simulink model "commrfsatlink"  (R2025a)
settings: Solver=VariableStepDiscrete  StartTime=0.0  StopTime=1  RelTol=1e-3  EnableMultiTasking=on
PreLoadFcn:
  | commrfsatlink_mask(1, 2, 1, 1, 1, ...
  |     0, 0, 0, 35600, 4000,[.4 .4],4,6,0,'No ADC');
values from neighbouring files (symbols this model uses):
  rfSatSourceSamplesPerSymbol = 400    [commrfsatlink_mask.m]
  rfSatSourceSampleTime = 1e-5    (= 1e-05)    [commrfsatlink_mask.m]
undefined symbols (not defined in the file or in its folder): paramRFSatLink, QAM
libraries: commrflib2 x6, dspsigops x3, commrfcorlib x2, dspsolvers x2, simulink x2, commfilt2 x2, commdigbbndam3 x2, commdemoslib x1, impairlib x1, commsink2 x1, commrandsrc3 x1, commsync2 x1
Description:
  | RF Satellite Link
settings Model: FPTRunName=Active  ExtModeAutoUpdateStatusClock=off  Creator=The MathWorks, Inc.  LastModifiedBy=daniel
settings SolverCC: AlgebraicLoopSolver=TrustRegion
settings DataIOCC: LimitDataPoints=on  SaveFormat=Array  SaveOutput=off  SaveTime=off  ReturnWorkspaceOutputs=off  SignalLoggingName=satlinkSigsOut
settings OptimizationCC: OptimizeBlockIOStorage=off  BufferReuse=off  GlobalBufferReuse=off  ExpressionFolding=off  ExpressionDepthLimit=2147483647.0  LocalBlockOutputs=off  InitFltsAndDblsToZero=on  EfficientMapNaN2IntZero=off  LifeSpan=inf  BufferReusableBoundary=off  OptimizeDataStoreBuffers=off  BusAssignmentInplaceUpdate=off
settings DebuggingCC: SaveWithParameterizedLinksMsg=none  UnderspecifiedInitializationDetection=Classic  MergeDetectMultiDrivingBlocksExec=none  CheckExecutionContextPreStartOutputMsg=on  SignalResolutionControl=TryResolveAllWithWarning  InheritedTsInSrcMsg=none  MultiTaskDSMMsg=warning  MultiTaskCondExecSysMsg=none  SigSpecEnsureSampleTimeMsg=none  FcnCallInpInsideContextMsg=warning  UnconnectedInputMsg=warning  UnconnectedOutputMsg=warning  UnconnectedLineMsg=warning  BusObjectLabelMismatch=none  AllowSymbolicDim=off  StateNameClashWarn=warning  PregeneratedLibrarySubsystemCodeDiagnostic=none  SFUnexpectedBacktrackingDiag=warning  SFNoUnconditionalDefaultTransitionDiag=warning  SFExecutionAtInitializationDiag=none  ArithmeticOperatorsInVariantConditions=warning
settings HardwareCC: ProdBitPerPointer=32.0  ProdLargestAtomicFloat=None  ProdIntDivRoundTo=Undefined  ProdEndianess=Unspecified  ProdWordSize=32.0  ProdHWDeviceType=32-bit Generic  TargetUnknown=on
settings ModelReferenceCC: UpdateModelReferenceTargets=IfOutOfDate  EnableRefExpFcnMdlSchedulingChecks=on  PropagateSignalLabelsOutOfModel=off
settings SFSimCC: SimUseLocalCustomCode=off  CustomCodeUndefinedFunction=UseInterfaceOnly
settings RTWCC: RTWUseLocalCustomCode=off  GPUComputeCapability=3.5
settings CodeAppCC: StateflowObjectComments=on
settings GRTTargetCC: TargetFcnLib=ansi_tfl_tmw.mat  TargetLangStandard=C89/C90 (ANSI)  CombineOutputUpdateFcns=off  GRTInterface=on
settings ConfigComp: CovMetricSettings=dw  CovSaveCumulativeToWorkspaceVar=on  CovSaveSingleToWorkspaceVar=on  CovExternalEMLEnable=off  CovSFcnEnable=off

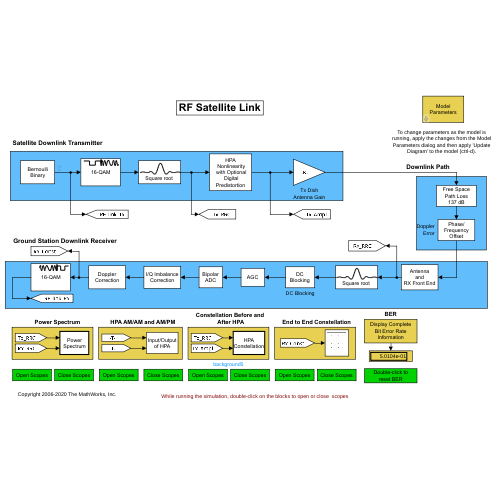
[thumbnail: Simulink's stored preview of the top-level diagram]
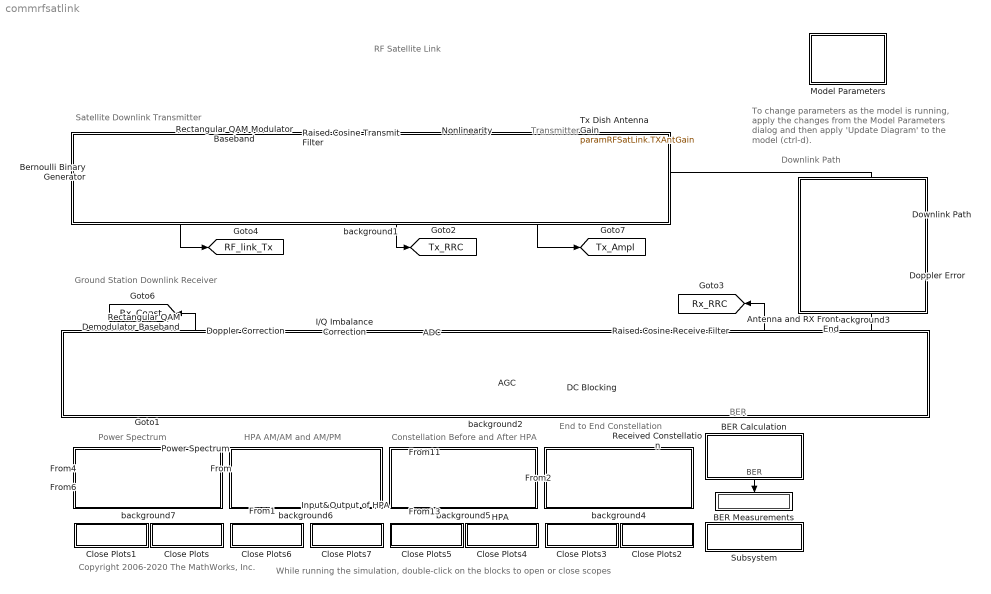
== system commrfsatlink ==
  note: Ground Station Downlink Receiver
  note: BER
  note: To change parameters as the model is running, apply the changes from the Model Parameters dialog and then apply 'Update Diagram' to the model (ctrl-d).
  note: RF Satellite Link
  note: Constellation Before and
      | After HPA
  note: Transmitter
  note: Power Spectrum
  note: While running the simulation, double-click on the blocks to open or close scopes
  note: Downlink Path
  note: End to End Constellation
  note: HPA AM/AM and AM/PM
  note: Copyright 2006-2020 The MathWorks, Inc.
  note: Satellite Downlink Transmitter
  ADC : Subsystem
      mask Display: disp('Bipolar\nADC')
  AGC : commrfcorlib/AGC  LegacyMode=off  DetectorMethod=Rectifier  LoopMethod=Linear  UpdatePeriod=100  StepSize=0.1  AdaptationStepSize=0.01  DesiredOutputPower=1  AveragingLength=256  MaximumGain=30  MaxPowerGain=400  GainOutputPort=off  InputPowerOutputPort=off  SimulateUsing=Code generation
  Antenna and RX Front End : Subsystem
      mask Display: disp('Antenna\nand\nRX Front End')
  BER Calculation : Subsystem
      mask Display: disp('Display Complete\nBit Error Rate\nInformation');
  BER Measurements : Display
      settings: Format=short_e
  Bernoulli Binary Generator : commrandsrc3/Bernoulli Binary Generator  ProbabilityOfZero=0.5  SeedSource=Parameter  Seed=37  SampleTime=rfSatSourceSampleTime  SamplesPerFrame=rfSatSourceSamplesPerSymbol  OutputDataType=double  SimulateUsing=Interpreted execution
  Close Plots : Subsystem
      settings: OpenFcn=|
      | sdspfscope2([],[],[],'ScopeUpdate',[bdroot '/Power Spectrum/Tx and Rx Spectrum'],'CloseFig');
      | set_param([bdroot '/Power Spectrum/Tx and Rx Spectrum'],'OpenScopeAtSimStart','off');
      mask Display: disp('Close Scopes');
  Close Plots1 : Subsystem
      settings: OpenFcn=|
      | sdspfscope2([],[],[],'ScopeUpdate',[bdroot '/Power Spectrum/Tx and Rx Spectrum'],'OpenFig');
      | set_param([bdroot '/Power Spectrum/Tx and Rx Spectrum'],'OpenScopeAtSimStart','on');
      mask Display: disp('Open Scopes');
  Close Plots2 : Subsystem
      settings: OpenFcn=|
      | sdspfscope2([],[],[],'ScopeUpdate',[bdroot '/Received Constellation'],'CloseFig');
      |    set_param([bdroot '/Received Constellation'],'OpenScopeAtSimStart','off');
      mask Display: disp('Close Scopes');
  Close Plots3 : Subsystem
      settings: OpenFcn=|
      | sdspfscope2([],[],[],'ScopeUpdate',[bdroot '/Received Constellation'],'OpenFig');
      |     set_param([bdroot '/Received Constellation'],'OpenScopeAtSimStart','on');
      mask Display: disp('Open Scopes');
  Close Plots4 : Subsystem
      settings: OpenFcn=|
      | sdspfscope2([],[],[],'ScopeUpdate',[bdroot '/HPA/RRC signal before and after HPA'],'CloseFig');
      |   set_param([bdroot '/HPA/RRC signal before and after HPA'],'OpenScopeAtSimStart','off');
      mask Display: disp('Close Scopes');
  Close Plots5 : Subsystem
      settings: OpenFcn=|
      | sdspfscope2([],[],[],'ScopeUpdate',[bdroot '/HPA/RRC signal before and after HPA'],'OpenFig');
      | set_param([bdroot '/HPA/RRC signal before and after HPA'],'OpenScopeAtSimStart','on');
      mask Display: disp('Open Scopes');
  Close Plots6 : Subsystem
      settings: OpenFcn=|
      | sdspfscope2([],[],[],'ScopeUpdate',[bdroot '/Input&Output of HPA/HPA AM to AM'],'OpenFig');
      | set_param([bdroot '/Input&Output of HPA/HPA AM to AM'],'OpenScopeAtSimStart','on');
      | sdspfscope2([],[],[],'ScopeUpdate',[bdroot '/Input&Output of HPA/HPA AM to PM'],'OpenFig');
      | set_param([bdroot '/Input&Output of HPA/HPA AM to PM'],'OpenScopeAtSimStart','on');
      mask Display: disp('Open Scopes');
  Close Plots7 : Subsystem
      settings: OpenFcn=|
      | sdspfscope2([],[],[],'ScopeUpdate',[bdroot '/Input&Output of HPA/HPA AM to AM'],'CloseFig');
      | set_param([bdroot '/Input&Output of HPA/HPA AM to AM'],'OpenScopeAtSimStart','off');
      | sdspfscope2([],[],[],'ScopeUpdate',[bdroot '/Input&Output of HPA/HPA AM to PM'],'CloseFig');
      | set_param([bdroot '/Input&Output of HPA/HPA AM to PM'],'OpenScopeAtSimStart','off');
      mask Display: disp('Close Scopes');
  DC Blocking : Subsystem
      mask Display: disp('DC\nBlocking')
  Doppler Correction : Subsystem
      mask Display: disp('Doppler\nCorrection')
  Doppler Error : commrflib2/Phase// Frequency Offset  phaseOffset=0  freqPort=off  freqOffset=paramRFSatLink.DoppOffset
  Downlink Path : commrflib2/Free Space Path Loss  mode=Distance and Frequency  dB=180  d=paramRFSatLink.Altitude  fc=paramRFSatLink.Frequency
  HPA : Subsystem  TreatAsAtomicUnit=on
      mask Display: disp('HPA\nConstellation')
  I/Q Imbalance Correction : Subsystem
      mask Display: disp('I/Q Imbalance\nCorrection')
  Input&Output of HPA : Subsystem
      mask Display: disp('Input/Output\nof HPA')
  Model Parameters : Subsystem  mask(Model Parameters){altitude=400, frequency=435, antDiam=[.5 .8], selTemp=500 (high noise level), selLvlBO=30 dB  (negligible nonlinearity), selDoppler=3 Hz, selNoPh=Negligible (-100 dBc/Hz @ 100 Hz), selImbal=None, selADC=High resolution (16 bits), selPreDistortion=off, selDcOffset=off, selCorrIQ=off, selCorrDoppler=on}
      mask prompts: altitude "Satellite altitude (km):"; frequency "Frequency (MHz):"; antDiam "Transmit and receive antenna diameters (m):"; selTemp "Noise temperature (K):"; selLvlBO "HPA backoff level:"; selDoppler "Doppler error:"; selNoPh "Phase noise:"; selImbal "I/Q imbalance and DC offset:"; selADC "ADC:"; selPreDistortion "Digital predistortion"; selDcOffset "DC offset correction"; selCorrIQ "I/Q imbalance correction"; selCorrDoppler "Doppler correction"
      mask help:
      | Select the scenarios from the mask to change the link parameters. Each of the mask parameters sets the parameters in the corresponding RF impairment or corresponding correction block(s).
      |
      | To make changes as the model is running, apply the changes from this dialog and then apply Update Diagram to the model (crtl-d).
      mask init:
      | commrfsatlink_mask(selLvlBO,selTemp, ...
      |     selDoppler, selImbal, selNoPh, ...
      |     selDcOffset, selCorrDoppler, selCorrIQ, altitude, ...
      |     frequency, antDiam,8,6,selPreDistortion,selADC);
      mask Help: helpview(commdhelp);
      mask TypeOptions selTemp: 0 (no noise) | 20 (very low noise level) | 290 (typical noise level) | 500 (high noise level)
      mask TypeOptions selLvlBO: 30 dB  (negligible nonlinearity) | 7 dB  (moderate nonlinearity) | 1 dB  (severe nonlinearity)
      mask TypeOptions selDoppler: 0 Hz | 3 Hz
      mask TypeOptions selNoPh: Negligible (-100 dBc/Hz @ 100 Hz) | Low  (-55 dBc/Hz @ 100 Hz) | High  (-48 dBc/Hz @ 100 Hz)
      mask TypeOptions selImbal: None | Amplitude imbalance (3 dB) | Phase imbalance (20 deg) | In-phase DC offset (1e-8) | Quadrature DC offset (5e-8)
      mask TypeOptions selADC: No ADC | High resolution (16 bits) | Medium resolution (8 bits) | Low resolution (3 bits)
      mask Display: disp('Model\nParameters');
  Nonlinearity : Subsystem
      mask Display: disp('HPA\n Nonlinearity\n with Optional\n Digital\nPredistortion')
  Power Spectrum : Subsystem  TreatAsAtomicUnit=on
      mask Display: disp('Power\nSpectrum')
  Raised Cosine Receive Filter : commfilt2/Raised Cosine Receive Filter  filtType=Square root  R=0.3  filtSpan=paramRFSatLink.FilterSpan  N=paramRFSatLink.SamplesPerSymbol  downFactor=paramRFSatLink.SamplesPerSymbol  downOffset=0  filterGain=1/sqrt(paramRFSatLink.SamplesPerSymbol)  InputProcessing=Columns as channels (frame based)  RateOptions=Enforce single-rate processing  framing=Mute  checkCoeff=off  variableName=rcRxFilt  currentFiltSpan=2*((2*(3))/2)  D=(2*(3))/2  inputOffset=0  sampMode=Mute  saveAsFlag=0  rateMode=Downsampling  checkGain=Normalized  launchFVT=off  roundingMode=Floor  overflowMode=off  coeffDataTypeStr=Inherit: Same word length as input  coeffMin=[]  coeffMax=[]  coeffLastDataTypeStr=Inherit: Same word length as input  accumDataTypeStr=Inherit: Same as product output  accumLastDataTypeStr=Inherit: Same as product output  outputDataTypeStr=Inherit: Same as accumulator  outputMin=[]  outputMax=[]  outputLastDataTypeStr=Inherit: Same as accumulator
  Raised Cosine Transmit Filter : commfilt2/Raised Cosine Transmit Filter  filtType=Square root  R=0.3  filtSpan=paramRFSatLink.SamplesPerSymbol  N=paramRFSatLink.SamplesPerSymbol  filterGain=sqrt(paramRFSatLink.SamplesPerSymbol)  InputProcessing=Columns as channels (frame based)  RateOptions=Enforce single-rate processing  framing=Mute  checkCoeff=off  variableName=rcTxFilt  checkGain=Normalized  sampMode=Mute  saveAsFlag=0  currentFiltSpan=2*((2*(3))/2)  D=(2*(3))/2  launchFVT=off  roundingMode=Floor  overflowMode=off  coeffDataTypeStr=Inherit: Same word length as input  coeffMin=[]  coeffMax=[]  coeffLastDataTypeStr=Inherit: Same word length as input  outputDataTypeStr=Inherit: Same as accumulator  outputMin=[]  outputMax=[]  outputLastDataTypeStr=Inherit: Same as accumulator
  Received Constellation : ConstellationDiagram  Tag=ScatterPlot  WindowPosition=[789.000000,1030.000000,270.000000,242.000000,]  ScopeFrameLocation=window  SamplesPerSymbol=8  SymbolsToDisplaySource=Property  SymbolsToDisplay=1000  ReferenceConstellation="[-0.94868+0.94868i -0.94868+0.31623i -0.94868-0.94868i -0.94868-0.31623i -0.31623+0.94868i -0.31623+0.31623i -0.31623-0.94868i -0.31623-0.31623i  0.94868+0.94868i  0.94868+0.31623i  0.94868-0.94868i  0.94868-0.31623i  0.31623+0.94868i  0.31623+0.31623i  0.31623-0.94868i  0.31623-0.31623i]"  Title=Received Constellation  XLimits=[-1.5 1.5]  YLimits=[-1.5 1.5]  AxesLimits=[-1.5 1.5]  ColorFading=on  DefaultConfigurationName=comm.scopes.ConstellationDiagramBlockCfg
  Rectangular QAM Demodulator Baseband : commdigbbndam3/Rectangular QAM Demodulator Baseband  M=16  OutType=Bit  DecType=Hard decision  VarSource=Dialog  Variance=1  Dec=Gray  Mapping=[0:15]  PowType=Average Power  MinDist=2  AvgPow=1  PeakPow=1  Ph=0  outDtype1=double  outDtype2=double  derotateFactorWordLen=16  derotateFactorDataTypeStr=Inherit: Same word length as input  derotateFactorLastDataTypeStr=Inherit: Same word length as input  denormFactorWordLen=16  denormFactorDataTypeStr=Inherit: Same word length as input  denormFactorLastDataTypeStr=Inherit: Same word length as input  prodOutWordLen=32  prodOutOverflowMode=Wrap  prodOutRoundingMode=Floor  prodOutOvFlMode=off  prodOutOvFlModeLastStrValue=off  sumWordLen=32
  Rectangular QAM Modulator Baseband : commdigbbndam3/Rectangular QAM Modulator Baseband  M=16  InType=Bit  Enc=Gray  Mapping=[0:15]  PowType=Average Power  MinDist=2  AvgPow=1  PeakPow=1  Ph=0  outDtype=double  outWordLen=16  outUDDataType=sfix(16)  outFracLenMode=Best precision  outFracLen=15  outDataTypeStr=double  outLastDataTypeStr=double
  Subsystem : Subsystem
      settings: OpenFcn=|
      | % Set value to reset BER
      | warning('off', 'Simulink:Engine:NonTunableVarChanged');
      | paramRFSatLink.resetBER = 1;
      | set_param(bdroot, 'SimulationCommand', 'update');
      | pause(0.1)
      | 
      | % Set value so that BER is not continually reset
      | paramRFSatLink.resetBER = 0;
      | set_param(bdroot, 'SimulationCommand', 'update');
      | warning('on', 'Simulink:Engine:NonTunableVarChanged');
      mask Display: disp('Double-click to\nreset BER')
  Tx Dish Antenna Gain : Gain  Gain=paramRFSatLink.TXAntGain  SaturateOnIntegerOverflow=on  OutDataTypeStr=Inherit: Same as input  ParamDataTypeStr=Inherit: Same as input
  background1 : Subsystem
      mask Display: disp('')
  background2 : Subsystem
      mask Display: disp('')
  background3 : Subsystem
      mask Display: disp('')
  background4 : Subsystem
      mask Display: disp('')
  background5 : Subsystem
      mask Display: disp('')
  background6 : Subsystem
      mask Display: disp('')
  background7 : Subsystem
      mask Display: disp('')
  tag scope: RF_link_Rx=global, RF_link_Tx=global, Rx_Const=global, Rx_RRC=global, Tx_Ampl=global, Tx_RRC=global
  wires:
  [HPA_In] -> Input&Output of HPA/1(In1)
  [HPA_Out] -> Input&Output of HPA/2(In2)
  Antenna and RX Front End/1(Out1) -> Raised Cosine Receive Filter/1, [Rx_RRC]
  [Rx_RRC] -> Power Spectrum/2(In2)
  Tx Dish Antenna Gain/1 -> Downlink Path/1
  [Tx_RRC] -> Power Spectrum/1(In1)
  Rectangular QAM Demodulator Baseband/1 -> [RF_link_Rx]
  [Rx_Const] -> Received Constellation/1
  Nonlinearity/1(Out2) -> [Tx_Ampl], Tx Dish Antenna Gain/1
  [Tx_Ampl] -> HPA/2(HPA Output)
  Raised Cosine Transmit Filter/1 -> [Tx_RRC], Nonlinearity/1(In)
  Doppler Correction/1(Out1) -> [Rx_Const], Rectangular QAM Demodulator Baseband/1
  [Tx_RRC] -> HPA/1(HPA Input)
  Doppler Error/1 -> Antenna and RX Front End/1(In1)
  I/Q Imbalance Correction/1(Out1) -> Doppler Correction/1(In1)
  Downlink Path/1 -> Doppler Error/1
  Rectangular QAM Modulator Baseband/1 -> Raised Cosine Transmit Filter/1
  Bernoulli Binary Generator/1 -> Rectangular QAM Modulator Baseband/1, [RF_link_Tx]
  BER Calculation/1(BER) -> BER Measurements/1
  Raised Cosine Receive Filter/1 -> DC Blocking/1(In1)
  DC Blocking/1(Out1) -> AGC/1
  AGC/1 -> ADC/1(In1)
  ADC/1(Out2) -> I/Q Imbalance Correction/1(In1)

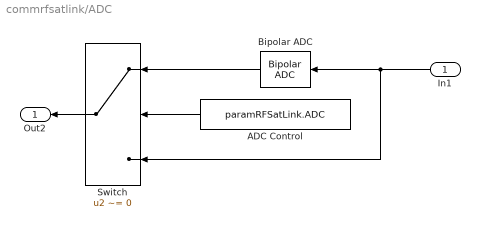
== system commrfsatlink/ADC ==
  In1 : Inport
  ADC Control : Constant  Value=paramRFSatLink.ADC  SampleTime=rfSatSourceSampleTime * rfSatSourceSamplesPerSymbol
  Bipolar ADC : commdemoslib/Bipolar ADC  FS_V=paramRFSatLink.ADC_VFS  N=paramRFSatLink.ADC_NumBits
  Switch : Switch  Criteria=u2 ~= 0  SaturateOnIntegerOverflow=off  InputSameDT=off
  Out2 : Outport  VectorParamsAs1DForOutWhenUnconnected=off
  wires:
  Bipolar ADC/1 -> Switch/1
  ADC Control/1 -> Switch/2
  In1/1 -> Bipolar ADC/1, Switch/3
  Switch/1 -> Out2/1

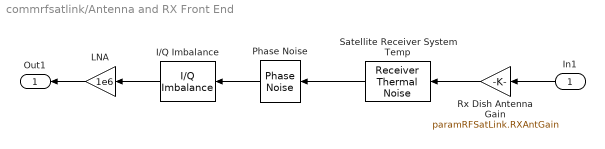
== system commrfsatlink/Antenna and RX Front End ==
  In1 : Inport
  I/Q Imbalance : commrflib2/I//Q Imbalance  ampImbal=paramRFSatLink.IQImbal(1)  phsImbal=paramRFSatLink.IQImbal(2)  Idc=paramRFSatLink.IQImbal(3)  Qdc=paramRFSatLink.IQImbal(4)
  LNA : Gain  Gain=1e6
  Phase Noise : impairlib/Phase Noise  Level=rfSatPhaseNoise  FrequencyOffset=100  SampleRate=2e5  RandomStream=mt19937ar with seed  Seed=2137  SimulateUsing=Interpreted execution
  Rx Dish Antenna Gain : Gain  Gain=paramRFSatLink.RXAntGain  SaturateOnIntegerOverflow=on  OutDataTypeStr=Inherit: Same as input  ParamDataTypeStr=Inherit: Same as input
  Satellite Receiver System Temp : commrflib2/Receiver Thermal Noise  LegacyMode=on  NoiseMethod=Noise temperature  NoiseTemperature=paramRFSatLink.RXTemp  NoiseFigure=20  NoiseFactor=2  Add290KAntennaNoise=off  ReferenceLoad=1  RandomStream=mt19937ar with seed  Seed=67987  SimulateUsing=Code generation
  Out1 : Outport  VectorParamsAs1DForOutWhenUnconnected=off
  wires:
  LNA/1 -> Out1/1
  Phase Noise/1 -> I/Q Imbalance/1
  Satellite Receiver System Temp/1 -> Phase Noise/1
  In1/1 -> Rx Dish Antenna Gain/1
  I/Q Imbalance/1 -> LNA/1
  Rx Dish Antenna Gain/1 -> Satellite Receiver System Temp/1

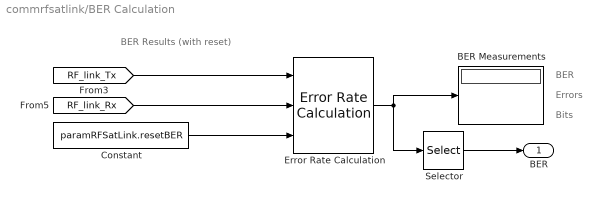
== system commrfsatlink/BER Calculation ==
  note: BER
  note: Errors
  note: Bits
  note: BER Results (with reset)
  BER Measurements : Display
  Constant : Constant  Value=paramRFSatLink.resetBER  SampleTime=rfSatSourceSampleTime * rfSatSourceSamplesPerSymbol
  Error Rate Calculation : commsink2/Error Rate Calculation  N=24  st_delay=0  cp_mode=Entire frame  subframe=[]  PMode=Port  WsName=ErrorVec  RsMode2=on  stop=off  numErr=200  maxBits=1e6
  Selector : Selector  InputPortWidth=3  IndexOptions=Index vector (dialog)  Indices=[1]  OutputSizes=1
  BER : Outport  VectorParamsAs1DForOutWhenUnconnected=off
  wires:
  [RF_link_Rx] -> Error Rate Calculation/2
  Error Rate Calculation/1 -> Selector/1, BER Measurements/1
  Constant/1 -> Error Rate Calculation/3
  Selector/1 -> BER/1
  [RF_link_Tx] -> Error Rate Calculation/1

== system commrfsatlink/Close Plots ==

== system commrfsatlink/Close Plots1 ==

== system commrfsatlink/Close Plots2 ==

== system commrfsatlink/Close Plots3 ==

== system commrfsatlink/Close Plots4 ==

== system commrfsatlink/Close Plots5 ==

== system commrfsatlink/Close Plots6 ==

== system commrfsatlink/Close Plots7 ==

== system commrfsatlink/DC Blocking ==
  In1 : Inport
  DC Blocker : dspsigops/DC Blocker  Algorithm=IIR  NormalizedBandwidth=0.0005  Length=8  Order=3  SimulateUsing=Code generation
  DC Blocker Control : Constant  Value=paramRFSatLink.DCBlock  SampleTime=rfSatSourceSampleTime * rfSatSourceSamplesPerSymbol
  Switch : Switch  Criteria=u2 > Threshold  SaturateOnIntegerOverflow=off  InputSameDT=off
  Out1 : Outport  VectorParamsAs1DForOutWhenUnconnected=off
  wires:
  In1/1 -> Switch/3, DC Blocker/1
  DC Blocker Control/1 -> Switch/2
  Switch/1 -> Out1/1
  DC Blocker/1 -> Switch/1

== system commrfsatlink/Doppler Correction ==
  In1 : Inport
  Carrier Synchronizer : commsync2/Carrier Synchronizer  Modulation=QAM  ModulationPhaseOffset=Auto  CustomPhaseOffset=0  SamplesPerSymbol=1  DampingFactor=0.707  NormalizedLoopBandwidth=0.001  EstimatedPhaseErrorOutputPort=off  SimulateUsing=Code generation
  Doppler Correction : Constant  Value=paramRFSatLink.CarrierSync  SampleTime=rfSatSourceSampleTime * rfSatSourceSamplesPerSymbol
  Switch : Switch  Criteria=u2 > Threshold  SaturateOnIntegerOverflow=off  InputSameDT=off
  Out1 : Outport  VectorParamsAs1DForOutWhenUnconnected=off
  wires:
  Doppler Correction/1 -> Switch/2
  Carrier Synchronizer/1 -> Switch/1
  Switch/1 -> Out1/1
  In1/1 -> Carrier Synchronizer/1, Switch/3

== system commrfsatlink/HPA ==
  HPA Input : Inport
  HPA Output : Inport  Port=2
  Matrix Concatenate : Concatenate  Mode=Multidimensional array  ConcatenateDimension=2
  RRC signal before and after HPA : ConstellationDiagram  WindowPosition=[177.000000,491.000000,1920.000000,977.000000,]  Visible=on  ScopeFrameLocation=window  SamplesPerSymbol=8  SymbolsToDisplaySource=Property  SymbolsToDisplay=1000  ReferenceConstellation=16-QAM  Title=RRC Signal Before and After HPA  XLimits=[-3.9233 3.9259]  YLimits=[-3.9233 3.9259]  AxesLimits=[-3.9233 3.9259]  ShowLegend=on  ShowReferenceConstellation=off  ColorFading=on  DefaultConfigurationName=comm.scopes.ConstellationDiagramBlockCfg
  wires:
  HPA Input/1 -> Matrix Concatenate/1
  HPA Output/1 -> Matrix Concatenate/2
  Matrix Concatenate/1 -> RRC signal before and after HPA/1

== system commrfsatlink/I//Q Imbalance Correction ==
  In1 : Inport
  I/Q Imbalance Compensator : commrfcorlib/I//Q Imbalance Compensator  CoefficientSource=Estimated from input signal  InitialCoefficient=0 + 0j  StepSizeSource=Property  StepSize=0.00001  AdaptInputPort=off  CoefficientOutputPort=off  SimulateUsing=Code generation
  I/Q Imbalance Correction : Constant  Value=paramRFSatLink.IQComp  SampleTime=rfSatSourceSampleTime * rfSatSourceSamplesPerSymbol
  Switch : Switch  Criteria=u2 > Threshold  SaturateOnIntegerOverflow=off  InputSameDT=off
  Out1 : Outport  VectorParamsAs1DForOutWhenUnconnected=off
  wires:
  I/Q Imbalance Correction/1 -> Switch/2
  I/Q Imbalance Compensator/1 -> Switch/1
  Switch/1 -> Out1/1
  In1/1 -> I/Q Imbalance Compensator/1, Switch/3

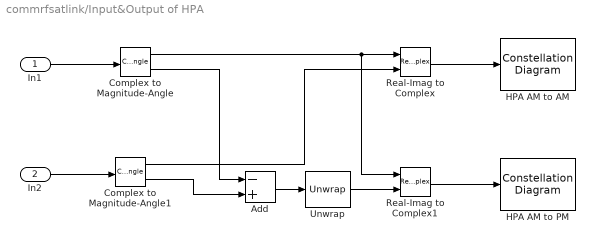
== system commrfsatlink/Input&Output of HPA ==
  In1 : Inport
  In2 : Inport  Port=2
  Add : Sum  Inputs=-+
  Complex to Magnitude-Angle : ComplexToMagnitudeAngle
  Complex to Magnitude-Angle1 : ComplexToMagnitudeAngle
  HPA AM to AM : ConstellationDiagram  Tag=ScatterPlot  WindowPosition=[1104 604 253 220]  SymbolsToDisplaySource=Property  SymbolsToDisplay=1000  Title=HPA AM to AM  XLimits=[-1.4713 6.1709]  YLimits=[-1.4713 6.1709]  AxesLimits=[-1.4713 6.1709]  XLabel=Input Amplitude  YLabel=Output Amplitude  ShowReferenceConstellation=off  ColorFading=on  DefaultConfigurationName=comm.scopes.ConstellationDiagramBlockCfg
      settings: OpenAtSimulationStart=off
  HPA AM to PM : ConstellationDiagram  Tag=ScatterPlot  WindowPosition=[842 605 253 220]  SymbolsToDisplaySource=Property  SymbolsToDisplay=1000  Title=HPA AM to PM  XLimits=[-1.0435 2.3201]  YLimits=[-1.0435 2.3201]  AxesLimits=[-1.0435 2.3201]  XLabel=Input Amplitude  YLabel=Phase Difference (rad)  ShowReferenceConstellation=off  ColorFading=on  DefaultConfigurationName=comm.scopes.ConstellationDiagramBlockCfg
      settings: OpenAtSimulationStart=off
  Real-Imag to Complex : RealImagToComplex
  Real-Imag to Complex1 : RealImagToComplex
  Unwrap : dspsigops/Unwrap  tol=pi  InputProcessing=Columns as channels (frame based)  running=on
  wires:
  Real-Imag to Complex/1 -> HPA AM to AM/1
  Complex to Magnitude-Angle1/1 -> Real-Imag to Complex/2
  Add/1 -> Unwrap/1
  In1/1 -> Complex to Magnitude-Angle/1
  In2/1 -> Complex to Magnitude-Angle1/1
  Real-Imag to Complex1/1 -> HPA AM to PM/1
  Unwrap/1 -> Real-Imag to Complex1/2
  Complex to Magnitude-Angle1/2 -> Add/2
  Complex to Magnitude-Angle/1 -> Real-Imag to Complex1/1, Real-Imag to Complex/1
  Complex to Magnitude-Angle/2 -> Add/1

== system commrfsatlink/Model Parameters ==

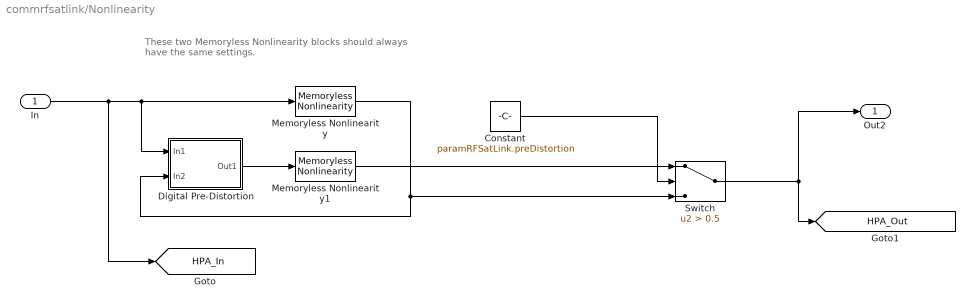
== system commrfsatlink/Nonlinearity ==
  note: These two Memoryless Nonlinearity blocks should always
      | have the same settings.
  In : Inport
  Constant : Constant  Value=paramRFSatLink.preDistortion  VectorParams1D=off  SampleTime=rfSatSourceSampleTime * rfSatSourceSamplesPerSymbol
  Digital Pre-Distortion : Subsystem
      mask Display: disp('Digital\nPredistortion')
  Memoryless Nonlinearity : commrflib2/Memoryless Nonlinearity  Model=saleh  Gain=0  Nonlinearity=OIP3  IIP3=30  OIP3=Inf  IP1dB=Inf  OP1dB=Inf  IPsat=Inf  OPsat=Inf  Table=[ -25, 5, -1; -10, 20, -2; 0, 27, 5; 5, 28, 12 ]  MagnitudeGainDB=0  Vsat=1  MagnitudeSmooth=0.5  PhaseGainRadian=-.45  PhaseSaturation=.88  PhaseSmooth=3.43  InputScaleDB=paramRFSatLink.GindB  AmAmParameters=[2.1587 1.1517]  AmPmParameters=[4.0330 9.1040]  OutputScaleDB=paramRFSatLink.GoutdB  ReferenceLoad=1  SimulateUsing=Code generation
  Memoryless Nonlinearity1 : commrflib2/Memoryless Nonlinearity  Model=saleh  Gain=0  Nonlinearity=OIP3  IIP3=30  OIP3=Inf  IP1dB=Inf  OP1dB=Inf  IPsat=Inf  OPsat=Inf  Table=[ -25, 5, -1; -10, 20, -2; 0, 27, 5; 5, 28, 12 ]  MagnitudeGainDB=0  Vsat=1  MagnitudeSmooth=0.5  PhaseGainRadian=-.45  PhaseSaturation=.88  PhaseSmooth=3.43  InputScaleDB=paramRFSatLink.GindB  AmAmParameters=[2.1587 1.1517]  AmPmParameters=[4.0330 9.1040]  OutputScaleDB=paramRFSatLink.GoutdB  ReferenceLoad=1  SimulateUsing=Code generation
  Switch : Switch  Criteria=u2 > Threshold  Threshold=0.5  ZeroCross=off  SaturateOnIntegerOverflow=off  InputSameDT=off
  Out2 : Outport  VectorParamsAs1DForOutWhenUnconnected=off
  tag scope: HPA_In=global, HPA_Out=global
  wires:
  Digital Pre-Distortion/1(Out1) -> Memoryless Nonlinearity1/1
  Memoryless Nonlinearity/1 -> Switch/3, Digital Pre-Distortion/2(In2)
  Switch/1 -> Out2/1, [HPA_Out]
  In/1 -> [HPA_In], Memoryless Nonlinearity/1, Digital Pre-Distortion/1(In1)
  Constant/1 -> Switch/2
  Memoryless Nonlinearity1/1 -> Switch/1

== system commrfsatlink/Power Spectrum ==
  In1 : Inport
  In2 : Inport  Port=2
  Matrix Concatenation : Concatenate  Mode=Multidimensional array  ConcatenateDimension=2
  Tx and Rx Spectrum : SpectrumAnalyzer  WindowPosition=[177.000000,491.000000,1920.000000,977.000000,]  Visible=on  ScopeFrameLocation=window  Method=Welch  SampleRate=200000  Span=200000  StartFrequency=-100000  StopFrequency=100000  AveragingMethod=Running  YLimits=[-100.6148 34.7731]  ShowLegend=on  ChannelNames="[\"Tramsitted \",\"Received\"]"  AllowFFTLengthLessThanSamplesPerUpdate=on  DefaultConfigurationName=spbscopes.SpectrumAnalyzerBlockCfg  IsFrequencyInputMode=0  FrequencyVectorPort=0  FrequencyVectorFromPort=0  FrequencyInputRBWPort=0  FrequencyInputRBWFromPort=0
  wires:
  In1/1 -> Matrix Concatenation/1
  In2/1 -> Matrix Concatenation/2
  Matrix Concatenation/1 -> Tx and Rx Spectrum/1

== system commrfsatlink/Subsystem ==

== system commrfsatlink/background1 ==

== system commrfsatlink/background2 ==

== system commrfsatlink/background3 ==

== system commrfsatlink/background4 ==

== system commrfsatlink/background5 ==

== system commrfsatlink/background6 ==

== system commrfsatlink/background7 ==

== system commrfsatlink/Nonlinearity/Digital Pre-Distortion ==
  In1 : Inport
  In2 : Inport  Port=2
  Distortion compensation : Subsystem
  Parameter Estimation : Subsystem
  Out1 : Outport  VectorParamsAs1DForOutWhenUnconnected=off
  wires:
  In2/1 -> Parameter Estimation/2(DUT Output)
  Distortion compensation/1(Pre-distorted Signal) -> Out1/1
  Parameter Estimation/2(d) -> Distortion compensation/2(d)
  Parameter Estimation/1(c) -> Distortion compensation/1(c)
  In1/1 -> Parameter Estimation/1(DUT Input), Distortion compensation/3(In)

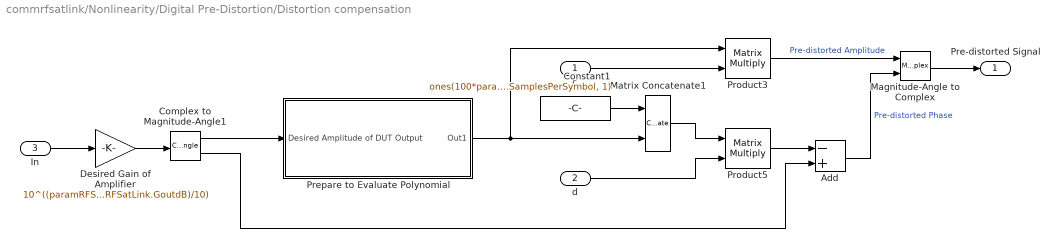
== system commrfsatlink/Nonlinearity/Digital Pre-Distortion/Distortion compensation ==
  c : Inport
  d : Inport  Port=2
  In : Inport  Port=3
  Add : Sum  Inputs=-+
  Complex to Magnitude-Angle1 : ComplexToMagnitudeAngle
  Constant1 : Constant  Value=ones(100*paramRFSatLink.SamplesPerSymbol, 1)
  Desired Gain of Amplifier : Gain  Gain=10^((paramRFSatLink.GindB + paramRFSatLink.GoutdB)/10)
  Magnitude-Angle to Complex : MagnitudeAngleToComplex
  Matrix Concatenate1 : Concatenate  Mode=Multidimensional array  ConcatenateDimension=2
  Prepare to Evaluate Polynomial : Subsystem
  Product3 : Product  Multiplication=Matrix(*)  RndMeth=Zero
  Product5 : Product  Multiplication=Matrix(*)  RndMeth=Zero
  Pre-distorted Signal : Outport  VectorParamsAs1DForOutWhenUnconnected=off
  wires:
  Constant1/1 -> Matrix Concatenate1/1
  Prepare to Evaluate Polynomial/1(Out1) -> Product3/1, Matrix Concatenate1/2
  Matrix Concatenate1/1 -> Product5/1
  Complex to Magnitude-Angle1/1 -> Prepare to Evaluate Polynomial/1(Desired Amplitude of DUT Output)
  Complex to Magnitude-Angle1/2 -> Add/2
  Magnitude-Angle to Complex/1 -> Pre-distorted Signal/1
  In/1 -> Desired Gain of Amplifier/1
  d/1 -> Product5/2
  Product3/1 -> Magnitude-Angle to Complex/1  "Pre-distorted Amplitude"
  Product5/1 -> Add/1
  Add/1 -> Magnitude-Angle to Complex/2  "Pre-distorted Phase"
  c/1 -> Product3/2
  Desired Gain of Amplifier/1 -> Complex to Magnitude-Angle1/1

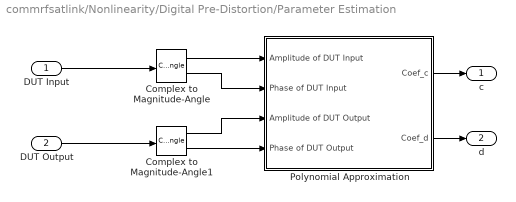
== system commrfsatlink/Nonlinearity/Digital Pre-Distortion/Parameter Estimation ==
  DUT Input : Inport
  DUT Output : Inport  Port=2
  Complex to Magnitude-Angle : ComplexToMagnitudeAngle
  Complex to Magnitude-Angle1 : ComplexToMagnitudeAngle
  Polynomial Approximation : Subsystem
  c : Outport  VectorParamsAs1DForOutWhenUnconnected=off
  d : Outport  Port=2  VectorParamsAs1DForOutWhenUnconnected=off
  wires:
  Complex to Magnitude-Angle/1 -> Polynomial Approximation/1(Amplitude of DUT Input)
  Complex to Magnitude-Angle1/2 -> Polynomial Approximation/4(Phase of DUT Output)
  Polynomial Approximation/2(Coef_d) -> d/1
  Polynomial Approximation/1(Coef_c) -> c/1
  Complex to Magnitude-Angle/2 -> Polynomial Approximation/2(Phase of DUT Input)
  Complex to Magnitude-Angle1/1 -> Polynomial Approximation/3(Amplitude of DUT Output)
  DUT Output/1 -> Complex to Magnitude-Angle1/1
  DUT Input/1 -> Complex to Magnitude-Angle/1

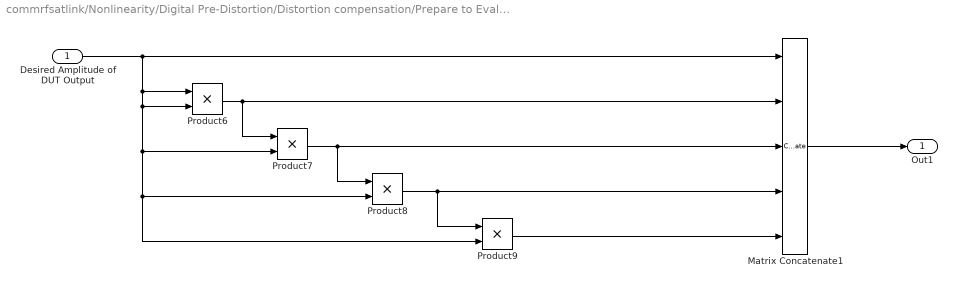
== system commrfsatlink/Nonlinearity/Digital Pre-Distortion/Distortion compensation/Prepare to Evaluate Polynomial ==
  Desired Amplitude of DUT Output : Inport
  Matrix Concatenate1 : Concatenate  NumInputs=5  Mode=Multidimensional array  ConcatenateDimension=2
  Product{6..9} (4 alike) : Product  RndMeth=Zero
  Out1 : Outport  VectorParamsAs1DForOutWhenUnconnected=off
  wires:
  Matrix Concatenate1/1 -> Out1/1
  Product9/1 -> Matrix Concatenate1/5
  Product8/1 -> Matrix Concatenate1/4, Product9/1
  Product6/1 -> Matrix Concatenate1/2, Product7/1
  Product7/1 -> Matrix Concatenate1/3, Product8/1
  Desired Amplitude of DUT Output/1 -> Matrix Concatenate1/1, Product6/1, Product6/2, Product7/2, Product8/2, Product9/2

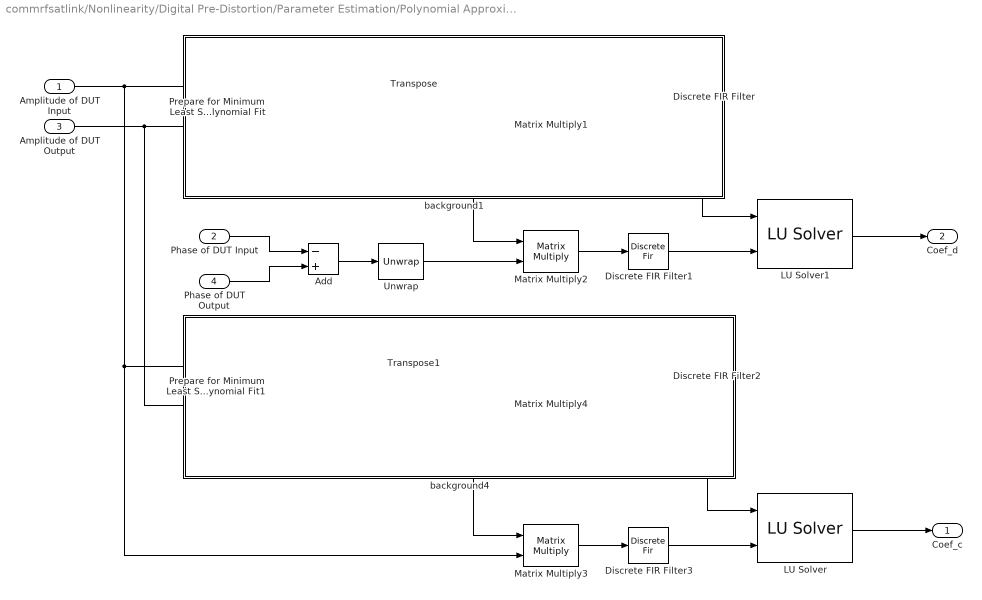
== system commrfsatlink/Nonlinearity/Digital Pre-Distortion/Parameter Estimation/Polynomial Approximation ==
  Amplitude of DUT Input : Inport
  Phase of DUT Input : Inport  Port=2
  Amplitude of DUT Output : Inport  Port=3
  Phase of DUT Output : Inport  Port=4
  Add : Sum  Inputs=-+
  Discrete FIR Filter{,1..3} (4 alike) : DiscreteFir  Coefficients=ones(1,50)  AccumDataTypeStr=Inherit: Same as product output
  LU Solver : dspsolvers/LU Solver
  LU Solver1 : dspsolvers/LU Solver
  Matrix Multiply{1..4} (4 alike) : Product  Multiplication=Matrix(*)
  Prepare for Minimum Least Square Error Polynomial Fit : Subsystem
  Prepare for Minimum Least Square Error Polynomial Fit1 : Subsystem
  Transpose : Math  Operator=transpose  SignedPower=on
  Transpose1 : Math  Operator=transpose  SignedPower=on
  Unwrap : dspsigops/Unwrap  tol=pi  InputProcessing=Columns as channels (frame based)  running=off
  background1 : Subsystem
      mask Display: disp('')
  background4 : Subsystem
      mask Display: disp('')
  Coef_c : Outport  VectorParamsAs1DForOutWhenUnconnected=off
  Coef_d : Outport  Port=2  VectorParamsAs1DForOutWhenUnconnected=off
  wires:
  Transpose/1 -> Matrix Multiply2/1, Matrix Multiply1/1
  LU Solver/1 -> Coef_c/1
  LU Solver1/1 -> Coef_d/1
  Phase of DUT Output/1 -> Add/2
  Discrete FIR Filter3/1 -> LU Solver/2
  Discrete FIR Filter/1 -> LU Solver1/1
  Discrete FIR Filter1/1 -> LU Solver1/2
  Amplitude of DUT Output/1 -> Prepare for Minimum Least Square Error Polynomial Fit/2(In2), Prepare for Minimum Least Square Error Polynomial Fit1/2(In2)
  Matrix Multiply2/1 -> Discrete FIR Filter1/1
  Unwrap/1 -> Matrix Multiply2/2
  Prepare for Minimum Least Square Error Polynomial Fit/1(Out1) -> Transpose/1, Matrix Multiply1/2
  Matrix Multiply3/1 -> Discrete FIR Filter3/1
  Matrix Multiply1/1 -> Discrete FIR Filter/1
  Amplitude of DUT Input/1 -> Matrix Multiply3/2, Prepare for Minimum Least Square Error Polynomial Fit1/1(In1), Prepare for Minimum Least Square Error Polynomial Fit/1(In1)
  Add/1 -> Unwrap/1
  Phase of DUT Input/1 -> Add/1
  Prepare for Minimum Least Square Error Polynomial Fit1/1(Out1) -> Transpose1/1, Matrix Multiply4/2
  Matrix Multiply4/1 -> Discrete FIR Filter2/1
  Transpose1/1 -> Matrix Multiply4/1, Matrix Multiply3/1
  Discrete FIR Filter2/1 -> LU Solver/1

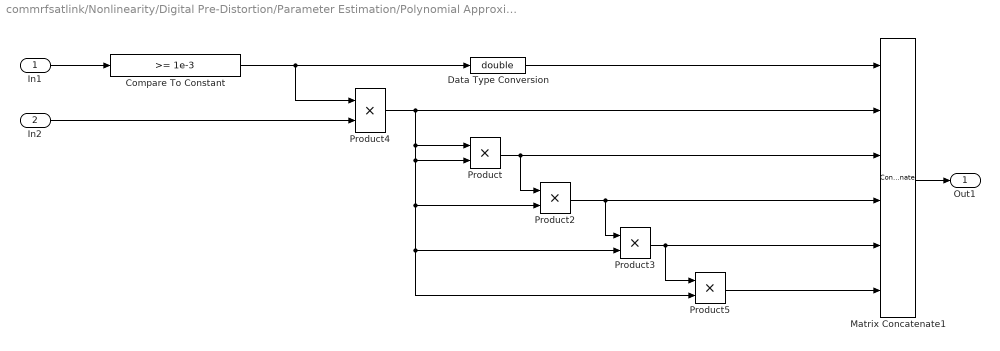
== system commrfsatlink/Nonlinearity/Digital Pre-Distortion/Parameter Estimation/Polynomial Approximation/Prepare for Minimum Least Square Error Polynomial Fit ==
  In1 : Inport
  In2 : Inport  Port=2
  Compare To Constant : simulink/Logic and Bit Operations/Compare To Constant  relop=>=  const=1e-3  OutDataTypeStr=uint8  ZeroCross=off
  Data Type Conversion : DataTypeConversion  OutDataTypeStr=double  SaturateOnIntegerOverflow=off  RndMeth=Floor
  Matrix Concatenate1 : Concatenate  NumInputs=6  Mode=Multidimensional array  ConcatenateDimension=2
  Product{,2..5} (5 alike) : Product  RndMeth=Zero
  Out1 : Outport  VectorParamsAs1DForOutWhenUnconnected=off
  wires:
  Data Type Conversion/1 -> Matrix Concatenate1/1
  In1/1 -> Compare To Constant/1
  Matrix Concatenate1/1 -> Out1/1
  Product5/1 -> Matrix Concatenate1/6
  Product4/1 -> Product/1, Product/2, Product2/2, Product3/2, Product5/2, Matrix Concatenate1/2
  Product/1 -> Matrix Concatenate1/3, Product2/1
  Product2/1 -> Matrix Concatenate1/4, Product3/1
  Product3/1 -> Matrix Concatenate1/5, Product5/1
  In2/1 -> Product4/2
  Compare To Constant/1 -> Data Type Conversion/1, Product4/1

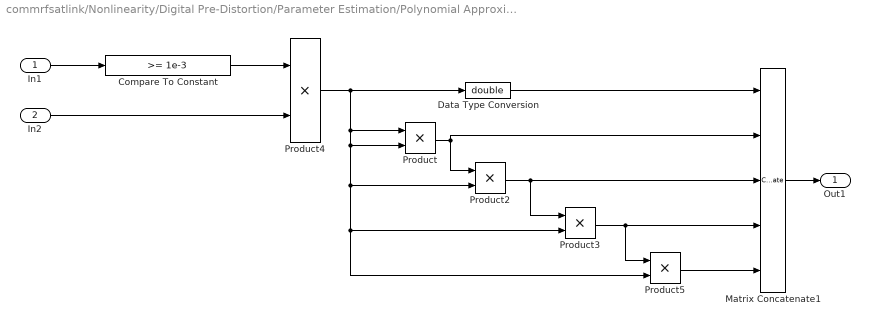
== system commrfsatlink/Nonlinearity/Digital Pre-Distortion/Parameter Estimation/Polynomial Approximation/Prepare for Minimum Least Square Error Polynomial Fit1 ==
  In1 : Inport
  In2 : Inport  Port=2
  Compare To Constant : simulink/Logic and Bit Operations/Compare To Constant  relop=>=  const=1e-3  OutDataTypeStr=uint8  ZeroCross=off
  Data Type Conversion : DataTypeConversion  OutDataTypeStr=double  SaturateOnIntegerOverflow=off  RndMeth=Floor
  Matrix Concatenate1 : Concatenate  NumInputs=5  Mode=Multidimensional array  ConcatenateDimension=2
  Product{,2..5} (5 alike) : Product  RndMeth=Zero
  Out1 : Outport  VectorParamsAs1DForOutWhenUnconnected=off
  wires:
  In1/1 -> Compare To Constant/1
  Matrix Concatenate1/1 -> Out1/1
  Product2/1 -> Product3/1, Matrix Concatenate1/3
  Product3/1 -> Product5/1, Matrix Concatenate1/4
  Product5/1 -> Matrix Concatenate1/5
  Product4/1 -> Product/1, Product/2, Product5/2, Product3/2, Product2/2, Data Type Conversion/1
  Product/1 -> Product2/1, Matrix Concatenate1/2
  In2/1 -> Product4/2
  Data Type Conversion/1 -> Matrix Concatenate1/1
  Compare To Constant/1 -> Product4/1

== system commrfsatlink/Nonlinearity/Digital Pre-Distortion/Parameter Estimation/Polynomial Approximation/background1 ==

== system commrfsatlink/Nonlinearity/Digital Pre-Distortion/Parameter Estimation/Polynomial Approximation/background4 ==
